simulink model "GaitMPC"  (R2023b)
settings: Solver=daessc  StartTime=0.0  StopTime=20  FixedStep=0.01  RelTol=1e-3
undefined symbols (not defined in the file or in its folder): dw_des, LFstates, LRstates, p_cur, p_des, px, py, pz, Q, RFstates, RRstates, v_cur, v_des, vx, vy, vz, w, w_des, X, Y, Z
libraries: sm_lib x57, nesl_utility x47
(part 3 of 3)

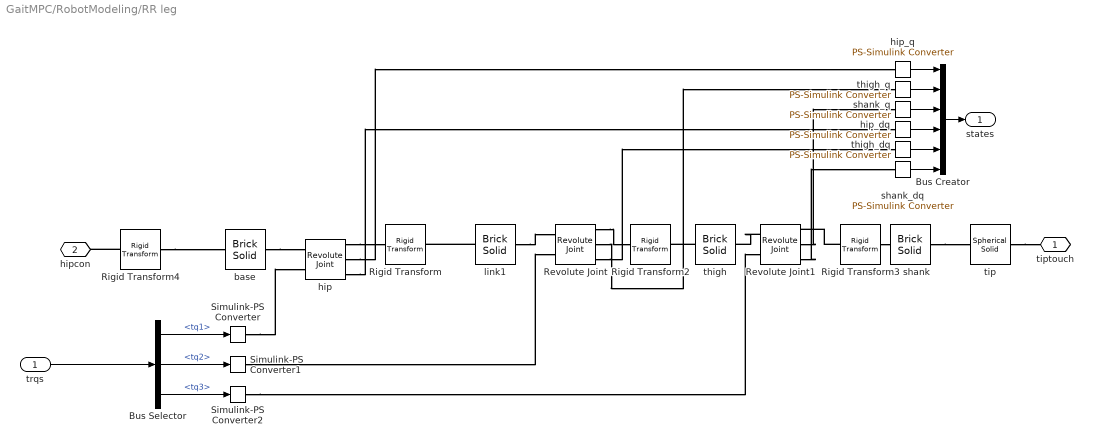
== system GaitMPC/RobotModeling/RR leg ==
  trqs : Inport
  Bus Creator : BusCreator  Inputs=6
  Bus Selector : BusSelector  OutputSignals=tq1,tq2,tq3
  Revolute Joint : sm_lib/Joints/Revolute Joint  JointMode=Normal  SenseConstraintForce=off  SenseConstraintForceX=off  SenseConstraintForceY=off  SenseConstraintForceZ=off  SenseConstraintTorque=off  SenseConstraintTorqueX=off  SenseConstraintTorqueY=off  SenseConstraintTorqueZ=off  SenseTotalForce=off  SenseTotalForceX=off  SenseTotalForceY=off  SenseTotalForceZ=off  SenseTotalTorque=off  SenseTotalTorqueX=off  SenseTotalTorqueY=off  SenseTotalTorqueZ=off  CompositeWrenchDir=FollowerOnBase  CompositeWrenchFrame=BaseFrame  EquilibriumPosition=0  EquilibriumPositionUnits=deg  SpringStiffness=0  SpringStiffnessUnits=N*m/deg  DampingCoefficient=0  DampingCoefficientUnits=N*m/(deg/s)  TorqueActuationMode=InputTorque  MotionActuationMode=ComputedMotion  SensePosition=on  SenseVelocity=on  SenseAcceleration=off  SenseTorqueForce=off  SenseLowerLimitTorqueForce=off  SenseUpperLimitTorqueForce=off  LowerLimitSpecify=off  LowerLimitBound=-90  LowerLimitBoundUnits=deg  LowerLimitStiffness=1e4  LowerLimitStiffnessUnits=N*m/deg  LowerLimitDamping=10  LowerLimitDampingUnits=N*m/(deg/s)  LowerLimitTransitionRegionWidth=0.1  LowerLimitTransitionRegionWidthUnits=deg  UpperLimitSpecify=off  UpperLimitBound=90  UpperLimitBoundUnits=deg  UpperLimitStiffness=1e4  UpperLimitStiffnessUnits=N*m/deg  UpperLimitDamping=10  UpperLimitDampingUnits=N*m/(deg/s)  UpperLimitTransitionRegionWidth=0.1  UpperLimitTransitionRegionWidthUnits=deg  PositionTargetSpecify=off  PositionTargetPriority=High  PositionTargetValue=0  PositionTargetValueUnits=deg  VelocityTargetSpecify=off  VelocityTargetPriority=High  VelocityTargetValue=0  VelocityTargetValueUnits=deg/s
  Revolute Joint1 : sm_lib/Joints/Revolute Joint  JointMode=Normal  SenseConstraintForce=off  SenseConstraintForceX=off  SenseConstraintForceY=off  SenseConstraintForceZ=off  SenseConstraintTorque=off  SenseConstraintTorqueX=off  SenseConstraintTorqueY=off  SenseConstraintTorqueZ=off  SenseTotalForce=off  SenseTotalForceX=off  SenseTotalForceY=off  SenseTotalForceZ=off  SenseTotalTorque=off  SenseTotalTorqueX=off  SenseTotalTorqueY=off  SenseTotalTorqueZ=off  CompositeWrenchDir=FollowerOnBase  CompositeWrenchFrame=BaseFrame  EquilibriumPosition=0  EquilibriumPositionUnits=deg  SpringStiffness=0  SpringStiffnessUnits=N*m/deg  DampingCoefficient=0  DampingCoefficientUnits=N*m/(deg/s)  TorqueActuationMode=InputTorque  MotionActuationMode=ComputedMotion  SensePosition=on  SenseVelocity=on  SenseAcceleration=off  SenseTorqueForce=off  SenseLowerLimitTorqueForce=off  SenseUpperLimitTorqueForce=off  LowerLimitSpecify=off  LowerLimitBound=-90  LowerLimitBoundUnits=deg  LowerLimitStiffness=1e4  LowerLimitStiffnessUnits=N*m/deg  LowerLimitDamping=10  LowerLimitDampingUnits=N*m/(deg/s)  LowerLimitTransitionRegionWidth=0.1  LowerLimitTransitionRegionWidthUnits=deg  UpperLimitSpecify=off  UpperLimitBound=90  UpperLimitBoundUnits=deg  UpperLimitStiffness=1e4  UpperLimitStiffnessUnits=N*m/deg  UpperLimitDamping=10  UpperLimitDampingUnits=N*m/(deg/s)  UpperLimitTransitionRegionWidth=0.1  UpperLimitTransitionRegionWidthUnits=deg  PositionTargetSpecify=off  PositionTargetPriority=High  PositionTargetValue=20  PositionTargetValueUnits=deg  VelocityTargetSpecify=off  VelocityTargetPriority=High  VelocityTargetValue=0  VelocityTargetValueUnits=deg/s
  Rigid Transform : sm_lib/Frames and Transforms/Rigid Transform  TranslationMethod=Cartesian  TranslationStandardOffset=0  TranslationStandardOffsetUnits=m  TranslationStandardAxis=+Z  TranslationCartesianOffset=[0.1 0 0]  TranslationCartesianOffsetUnits=m  TranslationROffset=0  TranslationROffsetUnits=m  TranslationZOffset=0  TranslationZOffsetUnits=m  TranslationThetaOffset=0  TranslationThetaOffsetUnits=deg  RotationMethod=None  RotationAngleUnits=deg  RotationStandardAxis=+Z  RotationAngle=0.0  RotationArbitraryAxis=[0 0 1]  FollAlignAxisA=+X  BaseAlignAxisA=+Y  FollAlignAxisB=+Y  BaseAlignAxisB=+Z  RotationSequenceAxes=FollowerAxes  RotationSequence=XYX  RotationSequenceAngles=[0 0 0]  RotationSequenceAnglesUnits=deg  RotationMatrix=[1 0 0; 0 1 0; 0 0 1]  Quaternion=[1 0 0 0]
  Rigid Transform2 : sm_lib/Frames and Transforms/Rigid Transform  TranslationMethod=Cartesian  TranslationStandardOffset=0  TranslationStandardOffsetUnits=m  TranslationStandardAxis=+Z  TranslationCartesianOffset=[0 -0.4 0]  TranslationCartesianOffsetUnits=m  TranslationROffset=0  TranslationROffsetUnits=m  TranslationZOffset=0  TranslationZOffsetUnits=m  TranslationThetaOffset=0  TranslationThetaOffsetUnits=deg  RotationMethod=None  RotationAngleUnits=deg  RotationStandardAxis=+Z  RotationAngle=0.0  RotationArbitraryAxis=[0 0 1]  FollAlignAxisA=+X  BaseAlignAxisA=+Y  FollAlignAxisB=+Y  BaseAlignAxisB=+Z  RotationSequenceAxes=FollowerAxes  RotationSequence=XYX  RotationSequenceAngles=[0 0 0]  RotationSequenceAnglesUnits=deg  RotationMatrix=[1 0 0; 0 1 0; 0 0 1]  Quaternion=[1 0 0 0]
  Rigid Transform3 : sm_lib/Frames and Transforms/Rigid Transform  TranslationMethod=Cartesian  TranslationStandardOffset=0  TranslationStandardOffsetUnits=m  TranslationStandardAxis=+Z  TranslationCartesianOffset=[0 -0.4 0]  TranslationCartesianOffsetUnits=m  TranslationROffset=0  TranslationROffsetUnits=m  TranslationZOffset=0  TranslationZOffsetUnits=m  TranslationThetaOffset=0  TranslationThetaOffsetUnits=deg  RotationMethod=None  RotationAngleUnits=deg  RotationStandardAxis=+Z  RotationAngle=0.0  RotationArbitraryAxis=[0 0 1]  FollAlignAxisA=+X  BaseAlignAxisA=+Y  FollAlignAxisB=+Y  BaseAlignAxisB=+Z  RotationSequenceAxes=FollowerAxes  RotationSequence=XYX  RotationSequenceAngles=[0 0 0]  RotationSequenceAnglesUnits=deg  RotationMatrix=[1 0 0; 0 1 0; 0 0 1]  Quaternion=[1 0 0 0]
  Rigid Transform4 : sm_lib/Frames and Transforms/Rigid Transform  TranslationMethod=Cartesian  TranslationStandardOffset=0  TranslationStandardOffsetUnits=m  TranslationStandardAxis=+Z  TranslationCartesianOffset=[0.35 0 1.25]  TranslationCartesianOffsetUnits=m  TranslationROffset=0  TranslationROffsetUnits=m  TranslationZOffset=0  TranslationZOffsetUnits=m  TranslationThetaOffset=0  TranslationThetaOffsetUnits=deg  RotationMethod=StandardAxis  RotationAngleUnits=deg  RotationStandardAxis=+Y  RotationAngle=90  RotationArbitraryAxis=[0 0 1]  FollAlignAxisA=+X  BaseAlignAxisA=+Y  FollAlignAxisB=+Y  BaseAlignAxisB=+Z  RotationSequenceAxes=FollowerAxes  RotationSequence=XYX  RotationSequenceAngles=[0 0 0]  RotationSequenceAnglesUnits=deg  RotationMatrix=[1 0 0; 0 1 0; 0 0 1]  Quaternion=[1 0 0 0]
  Simulink-PS Converter : nesl_utility/Simulink-PS Converter  PhysicalDomain=network_engine_domain  SubClassName=ps_input  LeftPortType=input  RightPortType=output  PseudoPeriodic=off  Frequencies=[]  NoiseDistribution=none  NoiseParameters=[]  Unit=1  AffineConversion=off  FilteringAndDerivatives=provide  SimscapeFilterOrder=1  InputFilterTimeConstant=0.001  UdotUserProvided=0
  Simulink-PS Converter1 : nesl_utility/Simulink-PS Converter  PhysicalDomain=network_engine_domain  SubClassName=ps_input  LeftPortType=input  RightPortType=output  PseudoPeriodic=off  Frequencies=[]  NoiseDistribution=none  NoiseParameters=[]  Unit=1  AffineConversion=off  FilteringAndDerivatives=provide  SimscapeFilterOrder=1  InputFilterTimeConstant=0.001  UdotUserProvided=0
  Simulink-PS Converter2 : nesl_utility/Simulink-PS Converter  PhysicalDomain=network_engine_domain  SubClassName=ps_input  LeftPortType=input  RightPortType=output  PseudoPeriodic=off  Frequencies=[]  NoiseDistribution=none  NoiseParameters=[]  Unit=1  AffineConversion=off  FilteringAndDerivatives=provide  SimscapeFilterOrder=1  InputFilterTimeConstant=0.001  UdotUserProvided=0
  base : sm_lib/Body Elements/Brick Solid  GraphicAmbientColor=[0.15 0.15 0.15 1.0]  BasedOnType=Density  BrickDimensions=[0.05 0.05 0.05]  BrickDimensionsUnits=m  CenterOfMass=[0 0 0]  CenterOfMassUnits=m  GraphicDiffuseColor=[0.0 0.8 0.8]  Density=1000  DensityUnits=kg/m^3  DoExposeReferenceFrame=on  GraphicEmissiveColor=[0.0 0.0 0.0 1.0]  ExportEntireGeometry=off  SerializedFrames=<Frames><Frame><Id>Frame1</Id><Value><Name>hip</Name><Origin><Source>GeometricFeature</Source><FeatureName>+z surface</FeatureName></Origin><PrimaryAxis><DefinedDirection>+Z</DefinedDirection><Source>ReferenceFrame</Source><SourceDirection>-X</SourceDirection><FeatureName></FeatureName></PrimaryAxis><SecondaryAxis><DefinedDirection>+X</DefinedDirection><Source>ReferenceFrame</Source><SourceDirection>+Z</SourceDirection><FeatureName></FeatureName></SecondaryAxis></Value></Frame></Frames>  MarkerShape=Sphere  MarkerSize=10  GraphicType=FromGeometry  InertiaType=CalculateFromGeometry  Mass=1  MassUnits=kg  MomentsOfInertia=[1 1 1]  MomentsOfInertiaUnits=kg*m^2  GraphicOpacity=1.0  ProductsOfInertia=[0 0 0]  ProductsOfInertiaUnits=kg*m^2  GraphicShininess=75  GraphicSpecularColor=[0.5 0.5 0.5 1.0]  GraphicVisPropType=SimpleVisualProperties
  hip : sm_lib/Joints/Revolute Joint  JointMode=Normal  SenseConstraintForce=off  SenseConstraintForceX=off  SenseConstraintForceY=off  SenseConstraintForceZ=off  SenseConstraintTorque=off  SenseConstraintTorqueX=off  SenseConstraintTorqueY=off  SenseConstraintTorqueZ=off  SenseTotalForce=off  SenseTotalForceX=off  SenseTotalForceY=off  SenseTotalForceZ=off  SenseTotalTorque=off  SenseTotalTorqueX=off  SenseTotalTorqueY=off  SenseTotalTorqueZ=off  CompositeWrenchDir=FollowerOnBase  CompositeWrenchFrame=BaseFrame  EquilibriumPosition=0  EquilibriumPositionUnits=deg  SpringStiffness=0  SpringStiffnessUnits=N*m/deg  DampingCoefficient=0  DampingCoefficientUnits=N*m/(deg/s)  TorqueActuationMode=InputTorque  MotionActuationMode=ComputedMotion  SensePosition=on  SenseVelocity=on  SenseAcceleration=off  SenseTorqueForce=off  SenseLowerLimitTorqueForce=off  SenseUpperLimitTorqueForce=off  LowerLimitSpecify=off  LowerLimitBound=-90  LowerLimitBoundUnits=deg  LowerLimitStiffness=1e4  LowerLimitStiffnessUnits=N*m/deg  LowerLimitDamping=10  LowerLimitDampingUnits=N*m/(deg/s)  LowerLimitTransitionRegionWidth=0.1  LowerLimitTransitionRegionWidthUnits=deg  UpperLimitSpecify=off  UpperLimitBound=90  UpperLimitBoundUnits=deg  UpperLimitStiffness=1e4  UpperLimitStiffnessUnits=N*m/deg  UpperLimitDamping=10  UpperLimitDampingUnits=N*m/(deg/s)  UpperLimitTransitionRegionWidth=0.1  UpperLimitTransitionRegionWidthUnits=deg  PositionTargetSpecify=off  PositionTargetPriority=High  PositionTargetValue=0  PositionTargetValueUnits=deg  VelocityTargetSpecify=off  VelocityTargetPriority=High  VelocityTargetValue=0  VelocityTargetValueUnits=deg/s
  hip_dq : nesl_utility/PS-Simulink Converter  PhysicalDomain=network_engine_domain  SubClassName=ps_output  LeftPortType=input  RightPortType=output  PseudoPeriodic=off  Frequencies=[]  VectorFormat=inherit  Unit=inherit  AffineConversion=off
  hip_q : nesl_utility/PS-Simulink Converter  PhysicalDomain=network_engine_domain  SubClassName=ps_output  LeftPortType=input  RightPortType=output  PseudoPeriodic=off  Frequencies=[]  VectorFormat=inherit  Unit=inherit  AffineConversion=off
  link1 : sm_lib/Body Elements/Brick Solid  GraphicAmbientColor=[0.15 0.15 0.15 1.0]  BasedOnType=Mass  BrickDimensions=[0.2 0.05 0.05]  BrickDimensionsUnits=m  CenterOfMass=[0 0 0]  CenterOfMassUnits=m  GraphicDiffuseColor=[0.5 0.5 0.5]  Density=1000  DensityUnits=kg/m^3  DoExposeReferenceFrame=on  GraphicEmissiveColor=[0.0 0.0 0.0 1.0]  ExportEntireGeometry=off  SerializedFrames=<Frames><Frame><Id>Frame1</Id><Value><Name>thigh</Name><Origin><Source>GeometricFeature</Source><FeatureName>+x surface</FeatureName></Origin><PrimaryAxis><DefinedDirection>+Z</DefinedDirection><Source>ReferenceFrame</Source><SourceDirection>+X</SourceDirection><FeatureName></FeatureName></PrimaryAxis><SecondaryAxis><DefinedDirection>+X</DefinedDirection><Source>ReferenceFrame</Source><SourceDirection>-Z</SourceDirection><FeatureName></FeatureName></SecondaryAxis></Value></Frame></Frames>  MarkerShape=Sphere  MarkerSize=10  GraphicType=FromGeometry  InertiaType=CalculateFromGeometry  Mass=0.2  MassUnits=kg  MomentsOfInertia=[1 1 1]  MomentsOfInertiaUnits=kg*m^2  GraphicOpacity=1.0  ProductsOfInertia=[0 0 0]  ProductsOfInertiaUnits=kg*m^2  GraphicShininess=75  GraphicSpecularColor=[0.5 0.5 0.5 1.0]  GraphicVisPropType=SimpleVisualProperties
  shank : sm_lib/Body Elements/Brick Solid  GraphicAmbientColor=[0.15 0.15 0.15 1.0]  BasedOnType=Mass  BrickDimensions=[0.07 0.8 0.07]  BrickDimensionsUnits=m  CenterOfMass=[0 0 0]  CenterOfMassUnits=m  GraphicDiffuseColor=[0.5 0.5 0.5]  Density=1000  DensityUnits=kg/m^3  DoExposeReferenceFrame=on  GraphicEmissiveColor=[0.0 0.0 0.0 1.0]  ExportEntireGeometry=off  SerializedFrames=<Frames><Frame><Id>Frame1</Id><Value><Name>F1</Name><Origin><Source>GeometricFeature</Source><FeatureName>-y surface</FeatureName></Origin><PrimaryAxis><DefinedDirection>+Z</DefinedDirection><Source>ReferenceFrame</Source><SourceDirection>+Z</SourceDirection><FeatureName></FeatureName></PrimaryAxis><SecondaryAxis><DefinedDirection>+X</DefinedDirection><Source>ReferenceFrame</Source><SourceDirection>+X</SourceDirection><FeatureName></FeatureName></SecondaryAxis></Value></Frame></Frames>  MarkerShape=Sphere  MarkerSize=10  GraphicType=FromGeometry  InertiaType=CalculateFromGeometry  Mass=0.5  MassUnits=kg  MomentsOfInertia=[1 1 1]  MomentsOfInertiaUnits=kg*m^2  GraphicOpacity=1.0  ProductsOfInertia=[0 0 0]  ProductsOfInertiaUnits=kg*m^2  GraphicShininess=75  GraphicSpecularColor=[0.5 0.5 0.5 1.0]  GraphicVisPropType=SimpleVisualProperties
  shank_dq : nesl_utility/PS-Simulink Converter  PhysicalDomain=network_engine_domain  SubClassName=ps_output  LeftPortType=input  RightPortType=output  PseudoPeriodic=off  Frequencies=[]  VectorFormat=inherit  Unit=inherit  AffineConversion=off
  shank_q : nesl_utility/PS-Simulink Converter  PhysicalDomain=network_engine_domain  SubClassName=ps_output  LeftPortType=input  RightPortType=output  PseudoPeriodic=off  Frequencies=[]  VectorFormat=inherit  Unit=inherit  AffineConversion=off
  thigh : sm_lib/Body Elements/Brick Solid  GraphicAmbientColor=[0.15 0.15 0.15 1.0]  BasedOnType=Mass  BrickDimensions=[0.07 0.8 0.07]  BrickDimensionsUnits=m  CenterOfMass=[0 0 0]  CenterOfMassUnits=m  GraphicDiffuseColor=[0.5 0.5 0.5]  Density=1000  DensityUnits=kg/m^3  DoExposeReferenceFrame=on  GraphicEmissiveColor=[0.0 0.0 0.0 1.0]  ExportEntireGeometry=off  SerializedFrames=<Frames><Frame><Id>Frame1</Id><Value><Name>F1</Name><Origin><Source>GeometricFeature</Source><FeatureName>-y surface</FeatureName></Origin><PrimaryAxis><DefinedDirection>+Z</DefinedDirection><Source>ReferenceFrame</Source><SourceDirection>+Z</SourceDirection><FeatureName></FeatureName></PrimaryAxis><SecondaryAxis><DefinedDirection>+Y</DefinedDirection><Source>ReferenceFrame</Source><SourceDirection>+Y</SourceDirection><FeatureName></FeatureName></SecondaryAxis></Value></Frame></Frames>  MarkerShape=Sphere  MarkerSize=10  GraphicType=FromGeometry  InertiaType=CalculateFromGeometry  Mass=0.5  MassUnits=kg  MomentsOfInertia=[1 1 1]  MomentsOfInertiaUnits=kg*m^2  GraphicOpacity=1.0  ProductsOfInertia=[0 0 0]  ProductsOfInertiaUnits=kg*m^2  GraphicShininess=75  GraphicSpecularColor=[0.5 0.5 0.5 1.0]  GraphicVisPropType=SimpleVisualProperties
  thigh_dq : nesl_utility/PS-Simulink Converter  PhysicalDomain=network_engine_domain  SubClassName=ps_output  LeftPortType=input  RightPortType=output  PseudoPeriodic=off  Frequencies=[]  VectorFormat=inherit  Unit=inherit  AffineConversion=off
  thigh_q : nesl_utility/PS-Simulink Converter  PhysicalDomain=network_engine_domain  SubClassName=ps_output  LeftPortType=input  RightPortType=output  PseudoPeriodic=off  Frequencies=[]  VectorFormat=inherit  Unit=inherit  AffineConversion=off
  tip : sm_lib/Body Elements/Spherical Solid  GraphicAmbientColor=[0.15 0.15 0.15 1.0]  BasedOnType=Mass  CenterOfMass=[0 0 0]  CenterOfMassUnits=m  GraphicDiffuseColor=[0.0 1.0 0.6]  Density=1000  DensityUnits=kg/m^3  DoExposeReferenceFrame=on  GraphicEmissiveColor=[0.0 0.0 0.0 1.0]  ExportEntireGeometry=on  SerializedExposedGeometries=<exposedGeometries><exposedGeom><rawGeomId>entire</rawGeomId><exposedGeomId>G</exposedGeomId></exposedGeom></exposedGeometries>  SerializedFrames=<Frames/>  MarkerShape=Sphere  MarkerSize=10  GraphicType=FromGeometry  InertiaType=CalculateFromGeometry  Mass=0.01  MassUnits=kg  MomentsOfInertia=[1 1 1]  MomentsOfInertiaUnits=kg*m^2  GraphicOpacity=1.0  ProductsOfInertia=[0 0 0]  ProductsOfInertiaUnits=kg*m^2  GraphicShininess=75  GraphicSpecularColor=[0.5 0.5 0.5 1.0]  SphereRadius=0.08  SphereRadiusUnits=m  GraphicVisPropType=SimpleVisualProperties
  tiptouch : PMIOPort  Side=Left
  hipcon : PMIOPort  Port=2  Side=Left
  states : Outport
  wires:
  Bus Creator/1 -> states/1
  Bus Selector/2 -> Simulink-PS Converter1/1  "<tq2>"
  thigh_q/1 -> Bus Creator/2
  thigh_dq/1 -> Bus Creator/5
  hip_q/1 -> Bus Creator/1
  Bus Selector/1 -> Simulink-PS Converter/1  "<tq1>"
  hip_dq/1 -> Bus Creator/4
  Bus Selector/3 -> Simulink-PS Converter2/1  "<tq3>"
  shank_dq/1 -> Bus Creator/6
  shank_q/1 -> Bus Creator/3
  trqs/1 -> Bus Selector/1
  connections:
  tip/LConn1 -- tiptouch/RConn1
  Revolute Joint1/RConn3 -- shank_dq/LConn1
  Revolute Joint1/RConn2 -- shank_q/LConn1
  Simulink-PS Converter2/RConn1 -- Revolute Joint1/LConn2
  Revolute Joint/RConn2 -- thigh_q/LConn1
  Simulink-PS Converter/RConn1 -- hip/LConn2
  hip/RConn3 -- hip_dq/LConn1
  base/LConn1 -- hip/LConn1
  hip/RConn1 -- Rigid Transform/LConn1
  Simulink-PS Converter1/RConn1 -- Revolute Joint/LConn2
  hip/RConn2 -- hip_q/LConn1
  link1/RConn1 -- Rigid Transform/RConn1
  Revolute Joint1/LConn1 -- thigh/LConn1
  Rigid Transform3/LConn1 -- Revolute Joint1/RConn1
  thigh/RConn1 -- Rigid Transform2/RConn1
  Rigid Transform3/RConn1 -- shank/RConn1
  Revolute Joint/RConn3 -- thigh_dq/LConn1
  Revolute Joint/RConn1 -- Rigid Transform2/LConn1
  Rigid Transform4/LConn1 -- hipcon/RConn1
  shank/LConn1 -- tip/RConn1
  Rigid Transform4/RConn1 -- base/RConn1
  link1/LConn1 -- Revolute Joint/LConn1

== matlab function GaitMPC/MPC-Controller/LegCoorProdunct2 ==
  data: t1 input; PLRx output; t2 input; t3 input
function PLRx = fcn(t1,t2,t3)
l1 = 0.2;
l2 = 0.8;
l3 = 0.8;

PBLR = [-1.25;0;-0.35];
%% 通过正运动学求出足端在腿坐标系中坐标
x = l1*cos(t1) - l3*(sin(t1)*sin(t2)*sin(t3) - cos(t2)*cos(t3)*sin(t1)) + l2*cos(t2)*sin(t1);
y = l3*(cos(t1)*sin(t2)*sin(t3) - cos(t1)*cos(t2)*cos(t3)) + l1*sin(t1) - l2*cos(t1)*cos(t2);
z = - l3*sin(t2 + t3) - l2*sin(t2);

PLR = [-z;y;x];
%% 转换到足端在机体坐标系中的坐标
PTLR = PBLR + PLR;

%% 转换成向量积矩阵
PLRx = [0 -PTLR(3) PTLR(2);
        PTLR(3) 0 -PTLR(1);
        -PTLR(2) PTLR(1) 0];

== matlab function GaitMPC/MPC-Controller/LegCoorProdunct3 ==
  data: t1 input; PLFx output; t2 input; t3 input
function PLFx = fcn(t1,t2,t3)
l1 = 0.2;
l2 = 0.8;
l3 = 0.8;

PBLF = [1.25;0;-0.35];
%% 通过正运动学求出足端在腿坐标系中坐标
x = l1*cos(t1) - l3*(sin(t1)*sin(t2)*sin(t3) - cos(t2)*cos(t3)*sin(t1)) + l2*cos(t2)*sin(t1);
y = l3*(cos(t1)*sin(t2)*sin(t3) - cos(t1)*cos(t2)*cos(t3)) + l1*sin(t1) - l2*cos(t1)*cos(t2);
z = - l3*sin(t2 + t3) - l2*sin(t2);

PLF = [-z;y;x];
%% 转换到足端在机体坐标系中的坐标
PTLF = PBLF + PLF;

%% 转换成向量积矩阵
PLFx = [0 -PTLF(3) PTLF(2);
        PTLF(3) 0 -PTLF(1);
        -PTLF(2) PTLF(1) 0];

== matlab function GaitMPC/MPC-Controller/Q2RotationMat ==
  data: Q input; Rsb output
function Rsb = Q2RotationMat(Q)
Q = Q';
Qang = Q(1);
Qang = max(min(Qang,0.99),-0.99);
theta = 2 * acos(Qang);
if theta == 0
    Rsb = eye(3);
else
    Omega = (Q(2:4)/sin(theta/2))';
    Rsb = [cos(theta) + Omega(1)^2*(1-cos(theta)),Omega(1)*Omega(2)*(1-cos(theta))-Omega(3)*sin(theta),Omega(1)*Omega(3)*(1-cos(theta))+Omega(2)*sin(theta);
       Omega(1)*Omega(2)*(1-cos(theta))+Omega(3)*sin(theta),cos(theta) + Omega(2)^2 * (1 - cos(theta)),Omega(2)*Omega(3)*(1-cos(theta))-Omega(1)*sin(theta);
       Omega(1)*Omega(3)*(1-cos(theta))-Omega(2)*sin(theta),Omega(2)*Omega(3)*(1-cos(theta))+Omega(1)*sin(theta),cos(theta) + Omega(3)^2 * (1 - cos(theta))];
end

== matlab function GaitMPC/MPC-Controller/MATLAB Function ==
  data: p_des input size=[3,1]; fRR1 output size=1; v_des input size=[3,1]; w_des input; dw_des input; p input size=[3,1]; v input; w input; dw input size=[3 1]; Rsb input; fRR2 output size=1; m input; Ib input; PRRx input; PRFx input; PLRx input; PLFx input; fRR3 output size=1; fRF1 output size=1; fRF2 output size=1; fRF3 output size=1; fLR1 output size=1; fLR2 output size=1; fLR3 output size=1; fLF1 output size=1; fLF2 output size=1; fLF3 output size=1
function [fRR1,fRR2,fRR3,fRF1,fRF2,fRF3,fLR1,fLR2,fLR3,fLF1,fLF2,fLF3]= MPCControl(p_des,v_des,w_des,dw_des,p,v,w,dw,Rsb,m,Ib,PRRx,PRFx,PLRx,PLFx)
% 定义状态空间方程
A = [zeros(3,3),eye(3),zeros(3,3),zeros(3,3),zeros(3,1);
     zeros(3,3),zeros(3,3),zeros(3,3),zeros(3,3),[0;-1;0];
     zeros(3,3),zeros(3,3),zeros(3,3),Rsb,zeros(3,1);
     zeros(3,3),zeros(3,3),zeros(3,3),zeros(3,3),zeros(3,1);
     zeros(1,13)];
B = [zeros(3,3),zeros(3,3),zeros(3,3),zeros(3,3);
     eye(3)/m,eye(3)/m,eye(3)/m,eye(3)/m;
     zeros(3,3),zeros(3,3),zeros(3,3),zeros(3,3);
     (Rsb*Ib*Rsb')*PRRx,(Rsb*Ib*Rsb')*PRFx,(Rsb*Ib*Rsb')*PLRx,(Rsb*Ib*Rsb')*PLFx;
     zeros(1,12)];

C = [eye(12),zeros(12,1)];
D = zeros(12,12);

% 离散化系统 采用某种近似离散化
T = 0.001;
% sys = ss(A,B,C,D);
% sys_d = c2d(sys,0.1);
A_k = T.*A + eye(13);
B_k = T * B;

% 定义权重矩阵
q = eye(13);
r = eye(12);

% 初始状态
x0 = [p;v;w;dw;10];
ref = [p_des;v_des;w_des;dw_des;10];
N_p = 5;
refs = repmat(ref,N_p,1); % 用于堆叠矩阵

% mpc求解
[m1, nA] = size(A_k);
[m2, n_in] = size(B_k);

%% calculate M
h = zeros(m1*N_p,nA);
M = zeros(m1*N_p,nA);
h(1:m1,:) = eye(m1);
M(1:m1,1:nA) = eye(m1) * A_k;

for kk = 2 : N_p
    h((kk - 1) * m1 + 1 : kk * m1, :) = h((kk - 2) * m1 + 1 : (kk - 1) * m1,:) * A_k;
    M((kk - 1) * m1 + 1 : kk * m1, :) = M((kk - 2) * m1 + 1 : (kk - 1) * m1, :) * A_k;
end

%% Calculate C
% first column of C
v = h * B_k;
THETA = zeros(N_p * m1, N_p * n_in);
THETA(:,1 : n_in) = v;

% Other columns of \Phi
for i = 2 : N_p
    THETA(:,(i-1) * n_in + 1 : i * n_in) = [zeros((i-1) * m1, n_in);v(1:(N_p - i + 1) * m1, 1 : n_in)];
end
    
    % Q,R
    % Q = [];
    % R = [];
    
    % for i = 1:N_p
    %     Q = blkdiag(Q, q);  % 从三个不同大小的矩阵创建一个分块对角矩阵
    %     R = blkdiag(R, r);  % 从三个不同大小的矩阵创建一个分块对角矩阵
    % end
    w = eye(65);
    R = eye(60);

H = 2 * ((THETA.')*w*THETA + R);
f = 2 * (THETA.')*w*(M*x0-refs);
options = optimoptions('quadprog','Algorithm','active-set');
res = quadprog(H, f, [],[],[],[],[],[],zeros(60,1),options);
res = res(1:12);

fRR1 = res(1)
fRR2 = res(2)
fRR3 = res(3)
fRF1 = res(4);
fRF2 = res(5);
fRF3 = res(6);
fLR1 = res(7);
fLR2 = res(8);
fLR3 = res(9);
fLF1 = res(10);
fLF2 = res(11);
fLF3 = res(12);

== matlab function GaitMPC/MPC-Controller/MATLAB Function1 ==
  data: ddp input size=[3 1]; ddw input size=[3 1]; fRR1 output size=1; m input; fRR2 output size=1; fRR3 output size=1; fRF1 output size=1; fRF2 output size=1; fRF3 output size=1; fLR1 output size=1; fLR2 output size=1; fLR3 output size=1; fLF1 output size=1; fLF2 output size=1; fLF3 output size=1; PRRx input; PRFx input; PLRx input; PLFx input; Rsb input; legStatus input
function [fRR1,fRR2,fRR3,fRF1,fRF2,fRF3,fLR1,fLR2,fLR3,fLF1,fLF2,fLF3] = SolveTipForces(ddp,ddw,m,PRRx,PRFx,PLRx,PLFx,Rsb,legStatus)
% g = [0;-10;0];
% 
% S = eye(6);
% W = diag(ones(1,12));
% 
% A = [eye(3),eye(3),eye(3),eye(3);
%      PRRx,PRFx,PLRx,PLFx];
% b = [m * (ddp + g);
%      Rsb*eye(3)*Rsb'*ddw];
% 
% %% 构建等式约束
% Aeq = zeros(12,12);
% beq = zeros(12,1);
% for num = 1:4
%     if legStatus(num) == 0
%         Aeq((num-1)*3+1:num*3,(num-1)*3+1:num*3) = eye(3);
%     end
% end
% options = optimoptions('quadprog','Algorithm','active-set');
% res = quadprog(A'*S*A + W,-b'*S*A,[],[],Aeq,beq,[],[],zeros(12,1),options);
% fRR1 = res(1);
% fRR2 = res(2);
% fRR3 = res(3);
% fRF1 = res(4);
% fRF2 = res(5);
% fRF3 = res(6);
% fLR1 = res(7);
% fLR2 = res(8);
% fLR3 = res(9);
% fLF1 = res(10);
% fLF2 = res(11);
% fLF3 = res(12);

== matlab function GaitMPC/Gait/MATLAB Function ==
  data: time input; legStatus output
function legStatus = Gait(time)
%% 一种步态的基本量
r = 0.5;
P = 0.6;
% 偏移时间遵循 RR RF LR LF 的顺序定义
legPhase = [0 P/2 P/2 0];
legStatus = [1 1 1 1]; % 1 stance;0 swing

if time <= 6
    legStatus = [1 1 1 1];
elseif mod(time,P) < P/2
    legStatus = [1 0 0 1];
else
    legStatus = [0 1 1 0];
end

== matlab function GaitMPC/MPC-Controller/Q2Euler ==
  data: Q input; w output
function w = Q2Euler(Q)
x = atan2(2*(Q(3)*Q(4)+Q(2)*Q(1)),1-2*(Q(2)^2+Q(4)^2));
y = atan2(2*(Q(2)*Q(4)+Q(3)*Q(1)),1-2*(Q(3)^2+Q(4)^2)); 
z = asin(2*(Q(4)*Q(1)-Q(2)*Q(3)));
w = [x;y;z];

== matlab function GaitMPC/Dynamic/RF Converter1 ==
  data: tq1 output size=1; fx input; fy input; fz input; t1 input; t2 input; t3 input; tq2 output size=1; tq3 output size=1
function [tq1,tq2,tq3]= forces2trqs(fx,fy,fz,t1,t2,t3)
Fx = fz;
Fy = fy;
Fz = -fx;
l1 = 0.2;
l2 = 0.8;
l3 = 0.8;
J = [l2*cos(t1)*cos(t2) - l1*sin(t1) - l3*(cos(t1)*sin(t2)*sin(t3) - cos(t1)*cos(t2)*cos(t3)), - l3*(cos(t2)*sin(t1)*sin(t3) + cos(t3)*sin(t1)*sin(t2)) - l2*sin(t1)*sin(t2), -l3*(cos(t2)*sin(t1)*sin(t3) + cos(t3)*sin(t1)*sin(t2));
l1*cos(t1) - l3*(sin(t1)*sin(t2)*sin(t3) - cos(t2)*cos(t3)*sin(t1)) + l2*cos(t2)*sin(t1),   l3*(cos(t1)*cos(t2)*sin(t3) + cos(t1)*cos(t3)*sin(t2)) + l2*cos(t1)*sin(t2),  l3*(cos(t1)*cos(t2)*sin(t3) + cos(t1)*cos(t3)*sin(t2));
                                                                                       0,                                                - l3*cos(t2 + t3) - l2*cos(t2),                                        -l3*cos(t2 + t3)];
tau = -J' * [Fx;Fy;Fz];
tq1 = tau(1);
tq2 = tau(2);
tq3 = tau(3);

== matlab function GaitMPC/Dynamic/RR Converter ==
  data: tq1 output size=1; fx input; fy input; fz input; t1 input; t2 input; t3 input; tq2 output size=1; tq3 output size=1
function [tq1,tq2,tq3]= forces2trqs(fx,fy,fz,t1,t2,t3)

Fx = fz;
Fy = fy;
Fz = -fx;
l1 = 0.2;
l2 = 0.8;
l3 = 0.8;
J = [l2*cos(t1)*cos(t2) - l1*sin(t1) - l3*(cos(t1)*sin(t2)*sin(t3) - cos(t1)*cos(t2)*cos(t3)), - l3*(cos(t2)*sin(t1)*sin(t3) + cos(t3)*sin(t1)*sin(t2)) - l2*sin(t1)*sin(t2), -l3*(cos(t2)*sin(t1)*sin(t3) + cos(t3)*sin(t1)*sin(t2));
l1*cos(t1) - l3*(sin(t1)*sin(t2)*sin(t3) - cos(t2)*cos(t3)*sin(t1)) + l2*cos(t2)*sin(t1),   l3*(cos(t1)*cos(t2)*sin(t3) + cos(t1)*cos(t3)*sin(t2)) + l2*cos(t1)*sin(t2),  l3*(cos(t1)*cos(t2)*sin(t3) + cos(t1)*cos(t3)*sin(t2));
                                                                                       0,                                                - l3*cos(t2 + t3) - l2*cos(t2),                                        -l3*cos(t2 + t3)];
tau = -J' * [Fx;Fy;Fz];
tq1 = tau(1);
tq2 = tau(2);
tq3 = tau(3);

== matlab function GaitMPC/Dynamic/LR Converter2 ==
  data: tq1 output size=1; fx input; fy input; fz input; t1 input; t2 input; t3 input; tq2 output size=1; tq3 output size=1
function [tq1,tq2,tq3]= forces2trqs(fx,fy,fz,t1,t2,t3)
isRight = -1;
Fx = isRight * fz;
Fy = fy;
Fz = -fx;
l1 = 0.2;
l2 = 0.8;
l3 = 0.8;
J = [l2*cos(t1)*cos(t2) - l1*sin(t1) - l3*(cos(t1)*sin(t2)*sin(t3) - cos(t1)*cos(t2)*cos(t3)), - l3*(cos(t2)*sin(t1)*sin(t3) + cos(t3)*sin(t1)*sin(t2)) - l2*sin(t1)*sin(t2), -l3*(cos(t2)*sin(t1)*sin(t3) + cos(t3)*sin(t1)*sin(t2));
l1*cos(t1) - l3*(sin(t1)*sin(t2)*sin(t3) - cos(t2)*cos(t3)*sin(t1)) + l2*cos(t2)*sin(t1),   l3*(cos(t1)*cos(t2)*sin(t3) + cos(t1)*cos(t3)*sin(t2)) + l2*cos(t1)*sin(t2),  l3*(cos(t1)*cos(t2)*sin(t3) + cos(t1)*cos(t3)*sin(t2));
                                                                                       0,                                                - l3*cos(t2 + t3) - l2*cos(t2),                                        -l3*cos(t2 + t3)];
tau = -J' * [Fx;Fy;Fz];
tq1 = tau(1);
tq2 = tau(2);
tq3 = tau(3);

== matlab function GaitMPC/Dynamic/LF Converter3 ==
  data: tq1 output size=1; fx input; fy input; fz input; t1 input; t2 input; t3 input; tq2 output size=1; tq3 output size=1
function [tq1,tq2,tq3]= forces2trqs(fx,fy,fz,t1,t2,t3)
isRight = -1;
Fx = isRight * fz;
Fy = fy;
Fz = isRight * -fx;
l1 = 0.2;
l2 = 0.8;
l3 = 0.8;
J = [l2*cos(t1)*cos(t2) - l1*sin(t1) - l3*(cos(t1)*sin(t2)*sin(t3) - cos(t1)*cos(t2)*cos(t3)), - l3*(cos(t2)*sin(t1)*sin(t3) + cos(t3)*sin(t1)*sin(t2)) - l2*sin(t1)*sin(t2), -l3*(cos(t2)*sin(t1)*sin(t3) + cos(t3)*sin(t1)*sin(t2));
l1*cos(t1) - l3*(sin(t1)*sin(t2)*sin(t3) - cos(t2)*cos(t3)*sin(t1)) + l2*cos(t2)*sin(t1),   l3*(cos(t1)*cos(t2)*sin(t3) + cos(t1)*cos(t3)*sin(t2)) + l2*cos(t1)*sin(t2),  l3*(cos(t1)*cos(t2)*sin(t3) + cos(t1)*cos(t3)*sin(t2));
                                                                                       0,                                                - l3*cos(t2 + t3) - l2*cos(t2),                                        -l3*cos(t2 + t3)];
tau = -J' * [Fx;Fy;Fz];
tq1 = tau(1);
tq2 = tau(2);
tq3 = tau(3);

== matlab function GaitMPC/MPC-Controller/LegCoorProdunct ==
  data: t1 input; PRRx output; t2 input; t3 input
function PRRx = fcn(t1,t2,t3)
l1 = 0.2;
l2 = 0.8;
l3 = 0.8;

PBRR = [-1.25;0;0.35];
%% 通过正运动学求出足端在腿坐标系中坐标
x = l1*cos(t1) - l3*(sin(t1)*sin(t2)*sin(t3) - cos(t2)*cos(t3)*sin(t1)) + l2*cos(t2)*sin(t1);
y = l3*(cos(t1)*sin(t2)*sin(t3) - cos(t1)*cos(t2)*cos(t3)) + l1*sin(t1) - l2*cos(t1)*cos(t2);
z = - l3*sin(t2 + t3) - l2*sin(t2);

PRR = [-z;y;x];
%% 转换到足端在机体坐标系中的坐标
PTRR = PBRR + PRR;

%% 转换成向量积矩阵
PRRx = [0 -PTRR(3) PTRR(2);
        PTRR(3) 0 -PTRR(1);
        -PTRR(2) PTRR(1) 0];

== matlab function GaitMPC/MPC-Controller/LegCoorProdunct1 ==
  data: t1 input; PRFx output; t2 input; t3 input
function PRFx = fcn(t1,t2,t3)
l1 = 0.2;
l2 = 0.8;
l3 = 0.8;

PBRF = [1.25;0;0.35];
%% 通过正运动学求出足端在腿坐标系中坐标
x = l1*cos(t1) - l3*(sin(t1)*sin(t2)*sin(t3) - cos(t2)*cos(t3)*sin(t1)) + l2*cos(t2)*sin(t1);
y = l3*(cos(t1)*sin(t2)*sin(t3) - cos(t1)*cos(t2)*cos(t3)) + l1*sin(t1) - l2*cos(t1)*cos(t2);
z = - l3*sin(t2 + t3) - l2*sin(t2);

PRF = [-z;y;x];
%% 转换到足端在机体坐标系中的坐标
PTRF = PBRF + PRF;

%% 转换成向量积矩阵
PRFx = [0 -PTRF(3) PTRF(2);
        PTRF(3) 0 -PTRF(1);
        -PTRF(2) PTRF(1) 0];
